simulink subsystem "ScaleU8Param"  (R2024a)
settings: Solver=VariableStepAuto  StartTime=0.0  StopTime=10.0  RelTol=1e-3
undefined symbols (not defined in the file or in its folder): max_midi_data
settings Model: Creator=dfurodet  LastModifiedBy=david

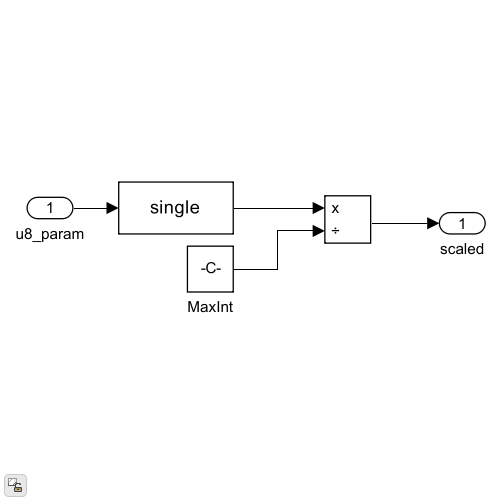
[thumbnail: Simulink's stored preview of the top-level diagram]
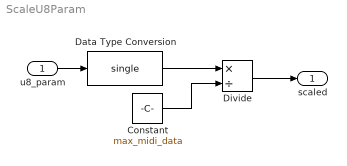
== system ScaleU8Param ==
  u8_param : Inport
  Constant : Constant  Value=max_midi_data  OutDataTypeStr=single
  Data Type Conversion : DataTypeConversion  OutDataTypeStr=single  SaturateOnIntegerOverflow=off  RndMeth=Floor
  Divide : Product  Inputs=*/
  scaled : Outport
  wires:
  Constant/1 -> Divide/2
  Data Type Conversion/1 -> Divide/1
  Divide/1 -> scaled/1
  u8_param/1 -> Data Type Conversion/1
